simulink model "model"  (R2018a)
settings: Solver=VariableStepAuto  StartTime=0.0  StopTime=10.0  RelTol=1e-3
undefined symbols (not defined in the file or in its folder): p
settings Model: Creator=mz-171742  LastModifiedBy=mz-171742

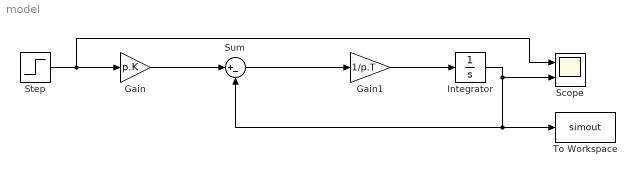
== system model ==
  Gain : Gain  Gain=p.K
  Gain1 : Gain  Gain=1/p.T
  Integrator : Integrator  InitialCondition=p.y0
  Scope : Scope  NumInputPorts=2
  Step : Step  Time=p.TStep  SampleTime=0
  Sum : Sum  Inputs=|+-
  To Workspace : ToWorkspace  VariableName=simout  SaveFormat=Structure With Time  SampleTime=-1
  wires:
  Gain1/1 -> Integrator/1
  Sum/1 -> Gain1/1
  Gain/1 -> Sum/1
  Step/1 -> Scope/1, Gain/1
  Integrator/1 -> Sum/2, To Workspace/1, Scope/2
